simulink model "linModel_S"  (R2021b)
settings: Solver=ode45  StartTime=0.0  StopTime=0.5  MaxStep=0.01  RelTol=1e-8
values from neighbouring files (symbols this model uses):
  A = [0 1; -k/mass-(4*C_magnetic*Ib^2)/(mass*gap^3) -c/mass]    [ex4.m]    (also in mp62.m = [-2 -3;-1 -4]; od.m = [0 1; -k/m-(4*C_magnetic*Ib^2)/(m*gap^3) -c/m])
  B = [0;(4*C_magnetic*Ib)/(mass*gap^2)]    [ex4.m]    (also in mp62.m = [0 1]'; od.m = [0;(4*C_magnetic*Ib)/(m*gap^2)])
  C = 0.0157    [ex2_1.m]    (also in ex3.m = 3.73e-06; ex4.m = [1 0]; mp62.m = [1 0]; od.m = [1 0;0 0])
  D = 0    [ex4.m]    (also in mp62.m; od.m)
settings Model: Creator=danli  LastModifiedBy=danli

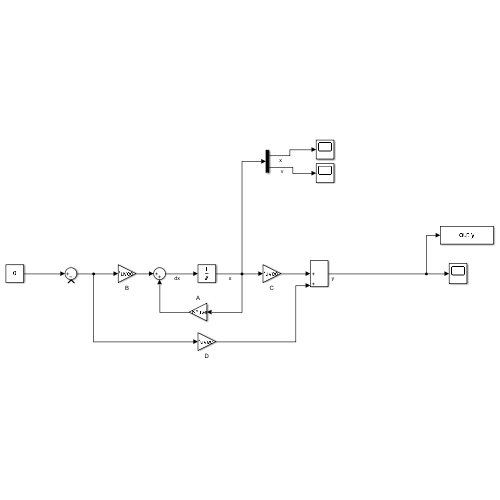
[thumbnail: Simulink's stored preview of the top-level diagram]
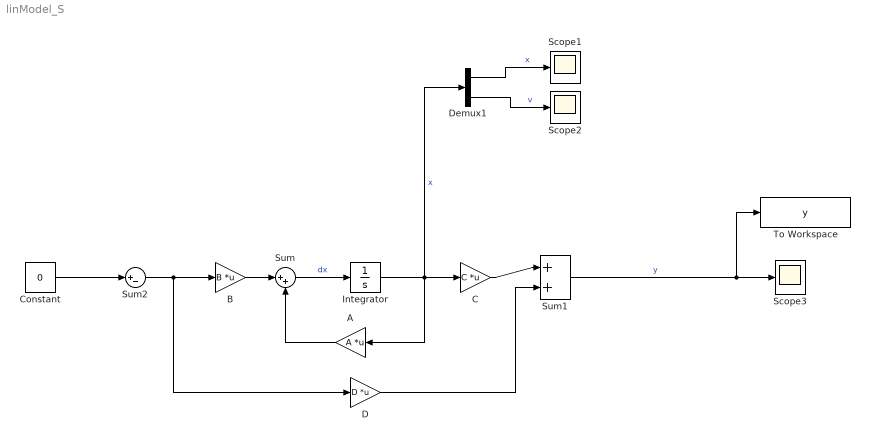
== system linModel_S ==
  A : Gain  Gain=A  Multiplication=Matrix(K*u) (u vector)
  B : Gain  Gain=B  Multiplication=Matrix(K*u) (u vector)
  C : Gain  Gain=C  Multiplication=Matrix(K*u) (u vector)
  Constant : Constant  Value=0
  D : Gain  Gain=D  Multiplication=Matrix(K*u) (u vector)
  Demux1 : Demux  Outputs=2
  Integrator : Integrator  InitialCondition=[5*10^-5 0]
  Scope1 : Scope
  Scope2 : Scope
  Scope3 : Scope
  Sum : Sum  Inputs=|++
  Sum1 : Sum  Inputs=||+|+
  Sum2 : Sum  Inputs=|+-
  To Workspace : ToWorkspace  VariableName=y  SaveFormat=Timeseries  SampleTime=-1
  wires:
  B/1 -> Sum/1
  A/1 -> Sum/2
  Sum/1 -> Integrator/1  "dx"
  Integrator/1 -> A/1, Demux1/1, C/1  "x"
  D/1 -> Sum1/2
  C/1 -> Sum1/1
  Sum2/1 -> B/1, D/1
  Constant/1 -> Sum2/1
  Demux1/1 -> Scope1/1  "x"
  Demux1/2 -> Scope2/1  "v"
  Sum1/1 -> To Workspace/1, Scope3/1  "y"
